simulink library "PCMULib"  (R2022b)
settings: Solver=ode45  StartTime=0.0  StopTime=10.0  RelTol=1e-3  EnableMultiTasking=on
undefined symbols (not defined in the file or in its folder): BreakpointData, BreakpointData1, BreakpointData2, BreakpointData_One_A, BreakpointData_Two_A, caaaa_dbi, caaaa_swi, cTmComprCtrl_n_i16SM4CmpHeatKiMax, cTmComprCtrl_n_i16SM4CmpHeatKiMin, cTmComprCtrl_n_i16SM4CmpHeatKpMax, cTmComprCtrl_n_i16SM4CmpHeatKpMin, cTmComprCtrl_Te_s32ErrCmpPIContinueHeatH, cTmComprCtrl_Te_s32ErrCmpPIContinueHeatL, cTmIn_n_ElacCmprReq_db, cTmIn_n_ElacCmprReq_sw, db, dbi, E2E_P01DataIDMode, E2E_P01ReceiverStatusType, EnumClass, iBit, initalValue, No_Runnable_Period, ObB_EidBsgStDerat_C, p_OVERRIDE_MASTER_SWITCH, SlDemoSign, sw, swi, SwitchOff_P, SwitchOn_P, Table, TableData_M, VCCTi33, VSysD_FidVehDerat1_C
libraries: simulink x22, CCMLib x11, simulink_need_slupdate x9, UXFD_Lib x7, canmsglib x2, PTCC_Lib x1, hdlsllib x1
(part 1 of 7)
settings Model: Creator=yaqi.zheng  LastModifiedBy=blue.ge
settings SolverCC: AlgebraicLoopSolver=TrustRegion
settings DataIOCC: LimitDataPoints=on  ReturnWorkspaceOutputs=off
settings OptimizationCC: LifeSpan=inf
settings DebuggingCC: UnconnectedInputMsg=warning  UnconnectedOutputMsg=warning  UnconnectedLineMsg=warning  AllowSymbolicDim=off  SFUnexpectedBacktrackingDiag=warning  SFNoUnconditionalDefaultTransitionDiag=warning  SFMachineParentedDataDiag=warning  ArithmeticOperatorsInVariantConditions=warning
settings ModelReferenceCC: EnableRefExpFcnMdlSchedulingChecks=on
settings SFSimCC: SimUseLocalCustomCode=off  CustomCodeUndefinedFunction=UseInterfaceOnly
settings RTWCC: RTWUseLocalCustomCode=off
settings CodeAppCC: StateflowObjectComments=on
settings GRTTargetCC: TargetLangStandard=C89/C90 (ANSI)
settings ConfigComp: CovMetricSettings=dw  CovSaveCumulativeToWorkspaceVar=on  CovSaveSingleToWorkspaceVar=on  CovExternalEMLEnable=off

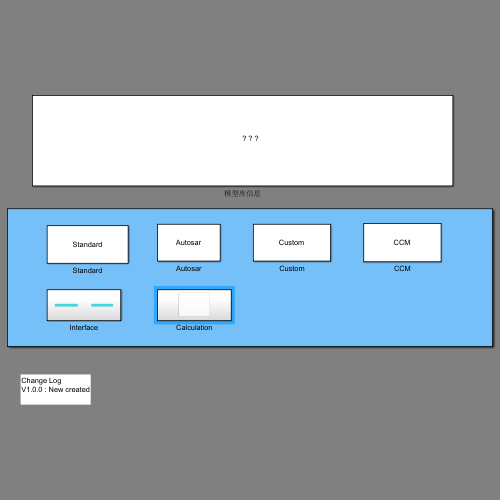
[thumbnail: Simulink's stored preview of the top-level diagram]
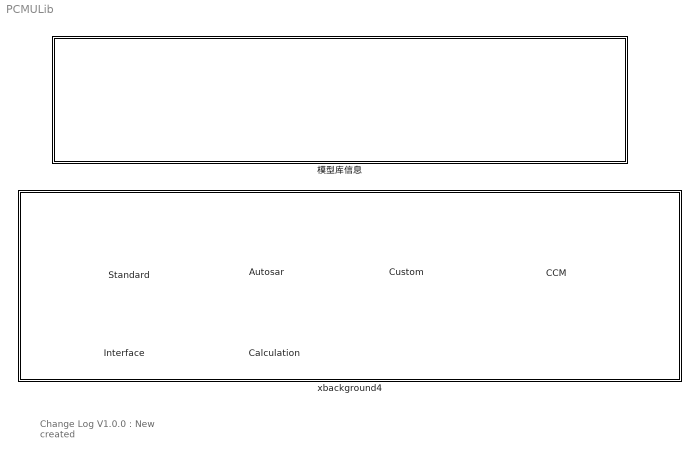
== system PCMULib ==
  note: Change Log
      | V1.0.0 : New created
  Autosar : Subsystem
      mask Display: disp('Autosar')
  CCM : Subsystem
      mask Display: disp('CCM')
  Calculation : Subsystem
  Custom : Subsystem
      mask Display: disp('Custom')
  Interface : Subsystem
  Standard : Subsystem
      mask Display: disp('Standard')
  xbackground4 : Subsystem
      mask Display: disp(' ')
  模型库信息 : Subsystem  mask(ModelHeader){prj=PCMU, desc=PCMU 模型库, ver=1.0.0, date=2023-10-11, rev=0, author=Blue, matlabver=MATLAB 2022b Version 9.13, simulinkver=MATLAB 2022b Version 10.6, stateflowver=MATLAB 2022b Version 10.7}
      mask prompts: prj "Project"; desc "Description"; ver "Version"; matlabver "MATLAB Ver"; simulinkver "Simulink Ver"; stateflowver "Stateflow Ver"
      mask init:
      | set_param(gcb, 'LinkStatus', 'none');
      mask Display:
      | plot([0 0 1 1 0],[0.03 1 1 0.03 0.03]) % 内层方框
      | plot([0.5 1],[0.85 0.85]) % 第一条横线
      | plot([0.5 1],[0.7 0.7]) % 第二条横线
      | plot([0.5 1],[0.55 0.55]) % 第三条线横线
      | plot([0.5 1],[0.4 0.4]) % 第四条线横线
      | plot([0 1],[0.25 0.25]) % 第五条横线
      | 
      | plot([0.5 0.5],[0.25 1]) % 第一条竖线
      | plot([0.60 0.60],[0.25 1])% 第二条竖线
      | plot([0.75 0.75],[0.25 1]) % 第三条竖线
      | plot([0.84 0.84],[0.25 1])% 第四条竖线
      | image(imread('geely.png','png'),[0.16 0.33 0.15 0.53]) % 图形位置
      | 
      | text(0.51,0.96,['\fontsize{8}\fontname{Times}\bfProject:'],'verticalAlignment','Top','horizontalAlignment','Left','texmode','on');
      | text(0.62,0.96,['\fontsize{8}\fontname{Times}\rm\fontsize{9}\fontsize{9}' prj],'verticalAlignment','Top','horizontalAlignment','Left','texmode','on');
      | 
      | text(0.51,0.81,['\fontsize{8}\fontname{Times}\bfVersion:' ],'verticalAlignment','Top','horizontalAlignment','Left','texmode','on');
      | text(0.62,0.81,['\fontsize{8}\fontname{Times}' ver],'verticalAlignment','Top','horizontalAlignment','Left','texmode','on');
      | 
      | text(0.51,0.67,['\fontsize{8}\fontname{Times}\bfDate:' ],'verticalAlignment','Top','horizontalAlignment','Left','texmode','on');
      | text(0.62,0.67,['\fontsize{8}\fontname{Times}\rm\fontsize{9}\fontsize{9}' date],'verticalAlignment','Top','horizontalAlignment','Left','texmode','on');
      | 
      | text(0.51,0.51,['\fontsize{8}\fontname{Times}\bfMATLAB Ver:' ],'verticalAlignment','Top','horizontalAlignment','Left','texmode','on');
      | text(0.62,0.51,['\fontsize{8}\fontname{Times}\rm\fontsize{9}\fontsize{9}' matlabver],'verticalAlignment','Top','horizontalAlignment','Left','texmode','on');
      | 
      | text(0.51,0.36,['\fontsize{8}\fontname{Times}\bfStateflow Ver:'],'verticalAlignment','Top','horizontalAlignment','Left','texmode','on');
      | text(0.62,0.36,['\fontsize{8}\fontname{Times}\rm\fontsize{9}\fontsize{9}' stateflowver],'verticalAlignment','Top','horizontalAlignment','Left','texmode','on');
      | %---------------------------------------------------------------------------------
      | text(0.76,0.96,['\fontsize{8}\fontname{Times}\bfAuthor:'],'verticalAlignment','Top','horizontalAlignment','Left','texmode','on');
      | text(0.86,0.96,['\fontsize{8}\fontname{Times}\rm\fontsize{9}\fontsize{9}' author],'verticalAlignment','Top','horizontalAlignment','Left','texmode','on');
      | 
      | text(0.76,0.81,['\fontsize{8}\fontname{Times}\bfRev:'],'verticalAlignment','Top','horizontalAlignment','Left','texmode','on');
      | text(0.86,0.81,['\fontsize{8}\fontname{Times}\rm\fontsize{9}\fontsize{9}' rev],'verticalAlignment','Top','horizontalAlignment','Left','texmode','on');
      | 
      | text(0.76,0.67,['\fontsize{8}\fontname{Times}\bfModel:'],'verticalAlignment','Top','horizontalAlignment','Left','texmode','on');
      | text(0.86,0.67,['\fontsize{8}\fontname{Times}\rm\fontsize{9}\fontsize{9}' desc],'verticalAlignment','Top','horizontalAlignment','Left','texmode','on');
      | 
      | text(0.76,0.51,['\fontsize{8}\fontname{Times}\bfSimulink Ver:'],'verticalAlignment','Top','horizontalAlignment','Left','texmode','on');
      | text(0.86,0.51,['\fontsize{8}\fontname{Times}\rm\fontsize{9}\fontsize{9}' simulinkver],'verticalAlignment','Top','horizontalAlignment','Left','texmode','on');
      | 
      | text(0.01,0.23,['\fontsize{8}\fontname{Times}\bfPROPRIETARY AND CONFIDENTIAL:\rm\fontsize{9}\newline\it\fontsize{10}\fontname{Arial}'                 'Geely Automobile Research Institute. All Right Reserved.'                 ],'verticalAlignment','Top','horizontalAlignment','Left','texmode','on');

== system PCMULib/Autosar ==
  note: Standard Core API AUTOSAR
  note: Advanced Core API AUTOSAR - use only if you know what you are doing
  note: E2E DEMO
  Constant6 : Constant  Value=72  OutDataTypeStr=Inherit: Inherit via back propagation
      settings: CopyFcn=set_param(gcbh,'ShowName','off');
  Constant7 : Constant  Value=220  OutDataTypeStr=Inherit: Inherit via back propagation
      settings: CopyFcn=set_param(gcbh,'ShowName','off');
  Dem_RepIUMPRDenLock : Subsystem  mask(Dem_RepIUMPRDenLock){}
      mask help: When enabled, this block will block the incrementation the denominator for Ratio Id Vc09XXXX.
      settings: AttributesFormatString=Dem_RepIUMPRDenLock
  Dem_RepIUMPRDenLock1 : PTCC_Lib/Autosar/Dem_RepIUMPRDenLock
      settings: AttributesFormatString=Dem_RepIUMPRDenLock
  Dem_RepIUMPRDenRelease : Subsystem  mask(Dem_RepIUMPRDenRelease){}
      mask help: When enabled, this block will release the incrementation the denominator for Ratio Id Vc09XXXX (i.e. if the conditions are fullfilled for incrementing the denominator for Ratio Id Vc09XXXX, it will be incremented).
      settings: AttributesFormatString=Dem_RepIUMPRDenRelease
  Dem_RepIUMPRFaultDetect : Subsystem  mask(Dem_RepIUMPRFaultDetect){}
      mask help: When enabled, report to the Core BSW, that Ratio Id Vc09XXXX has been able to detect a fault (increment Numerator for Ratio Id Vc09XXXX)
      settings: AttributesFormatString=Dem_RepIUMPRFaultDetect
  Dem_SetDTR : Subsystem  Description="API method to update mode $06 testdata.                                       Dem_SetDTR(UInt16 DTRId, sint32 TestVal, sint32 LowerLimit, sint32  UpperLimit, Ctrlval )"  mask(Vcc_SetDTR){lsb=1.0, offset=0}
      mask help:
      | Reports a DTR result with lower and upper limit.
      | The types of the TestValue and it limits should be Float32.
      | The test value and test limits are converted to Int32s using the
      | lsb and offset parameters in this block
      |
      | API is needed in OBD-relevant ECUs only
      settings: AttributesFormatString=Vcc_SetDTR
  Dem_SetEventStatusDepPF : Subsystem  TreatAsAtomicUnit=on  mask(Dem_SetEventStatusDepPre-Failed){}
      mask help:
      | Only to be used by dependability functions.
      | When enabled, events with status Pre-Failed is sent to the Diagnostic Core
      settings: AttributesFormatString=Dem_SetEventStatusDep\nPre-Failed
  Dem_SetEventStatusDepPP : Subsystem  TreatAsAtomicUnit=on  mask(Dem_SetEventStatusDepPre-Passed){}
      mask help:
      | Only to be used by dependability functions.
      | When enabled, events with status Pre-Passed is sent to the Diagnostic Core
      settings: AttributesFormatString=Dem_SetEventStatusDep\nPre-Passed
  Dem_SetEventStatusF : Subsystem  TreatAsAtomicUnit=on  mask(Dem_SetEventStatusFailed){}
      mask help: When enabled, events with status Failed is sent to the Diagnostic Core
      settings: AttributesFormatString=Dem_SetEventStatus\nFailed
  Dem_SetEventStatusP : Subsystem  mask(Dem_SetEventStatusPassed){}
      mask help: When enabled, events with status Passed is sent to the Diagnostic Core
      settings: AttributesFormatString=Dem_SetEventStatus\nPassed
  Dem_SetEventStatusPF : Subsystem  mask(Dem_SetEventStatusPre-Failed){}
      mask help: When enabled, events with status Pre-Failed is sent to the Diagnostic Core
      settings: AttributesFormatString=Dem_SetEventStatus\nPre-Failed
  Dem_SetEventStatusPP : Subsystem  mask(Dem_SetEventStatusPre-Passed){}
      mask help: When enabled, events with status Pre-Passed is sent to the Diagnostic Core
      settings: AttributesFormatString=Dem_SetEventStatus\nPre-Passed
  E2E_P01Protect : Subsystem
  E2E_P01_Check : Subsystem
  FiM_GetFunctionPermission : Subsystem  mask(FiM_GetFunctionPermission){}
      mask help:
      | When enabled, this block ask the core for permission to execute a monitor with the FID.
      | Note: If this is used for activating reconfigurations, Perm == 0 => Activate reconfiguration.
      settings: AttributesFormatString=FiM_GetFunctionPermission
  NamedConstant : Subsystem  mask(NamedConstant){const_name=VcEvName}
      mask prompts: const_name "Constant Name"
      mask help:
      | Enter a name for a preprocessor defined constant.
      | The following naming convention shall be used:
      | These prefixes shall be used for the following IDs (without underscores):
      | VcEv - Event IDs
      | VcFi - Function IDs (FiD)
      | VcRv - Ranking Value IDs
      | Vc06 - Mode $06 Test result IDs
      | Vc09 - IU(M)PR IDs (Mode $09)
      |
      | E.g.
      | VcEvBoostHigh - An event ID name for too high boost pressure
      | VcFiBoostPeak - A FiD for the Peak pressure boost monitor
      settings: AttributesFormatString=Named Constant
      mask Display: text(0.5, 0.5, get_param(gcb, 'const_name'), 'horizontalAlignment', 'center')
  Terminator7 : Terminator
  xbackground1 : UXFD_Lib/Autosar/xbackground4  SystemSampleTime=-1  VariantActivationTime=update diagram  Latency=0  AutoFrameSizeCalculation=off
  xbackground4 : Subsystem
      mask Display: disp(' ')
  xbackground5 : Subsystem
      mask Display: disp(' ')
  wires:
  E2E_P01Protect/1(E2E_P01Protect_ReturnType) -> Terminator7/1
  Constant6/1 -> E2E_P01Protect/1(DataLength)
  Constant7/1 -> E2E_P01Protect/2(DataID)

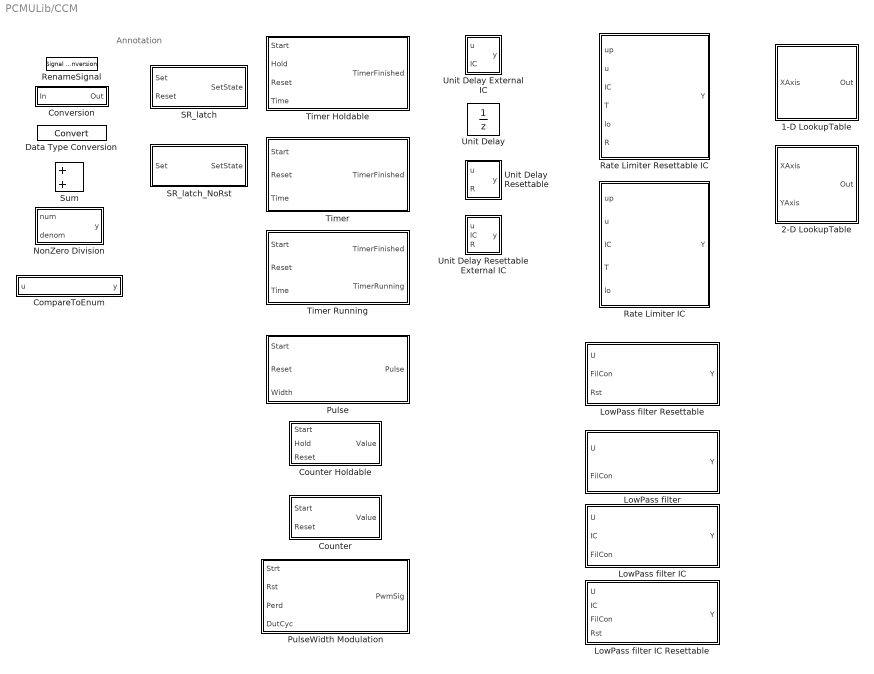
== system PCMULib/CCM ==
  note: Annotation
  1-D LookupTable : Subsystem  mask(1D Lookup table NGCC v1.1){TableData=[4 7 6], TableDataDataType=Inherit: auto, BreakpointsXAxis=[1:3], BreakpointsXAxisDataType=Inherit: auto}
      mask help:
      | NGCC version of the Simulink standard 2-D lookup table.
      | "X-axis" is used as notation instead of "breakpoints 1".
      | Deviation from standard 2-D lookup table default settings:
      | - Extrapolation method: Clip, use last table value for inputs at or above last breakpoint.
      | - Saturate on integer overflow.
      | - Integer rounding mode: Floor
      | - Does NOT require all inputs to have the same data type
      |
      | Mx-VDev tested: Yes
      mask init:
      | blkNameMask = gcb;
      | 
      | % Redraw block at resize
      | set_param(blkNameMask,'MaskRunInitForIconRedraw','on')
      mask Display:
      | pos = get_param(gcb, 'Position');
      | width = pos(3) - pos(1);
      | height = pos(4) - pos(2);
      | doPlot = true;
      | blockHandle = gcb;
      | try
      |     tableDialogText = get_param(blockHandle,'TableData');
      |     try
      |         table = evalin('base',tableDialogText);
      |         tableValue = table.Value;
      |     catch
      |         tableValue = recursiveMaskParameterSearch(blockHandle,tableDialogText);
      |     end
      |     breakpointsXAxisDialogText = get_param(blockHandle,'BreakpointsXAxis');
      |     try
      |         breakpointsXAxisHandle = evalin('base',breakpointsXAxisDialogText);
      |         bp1 = breakpointsXAxisHandle.Value;
      |     catch
      |         bp1 = recursiveMaskParameterSearch(blockHandle,breakpointsXAxisDialogText);
      |     end
      | catch
      |     tableValue = str2num(get_param(blockHandle,'TableData'));
      |     bp1 = str2num(get_param(blockHandle,'BreakpointsXAxis'));
      |     doPlot = true;
      |     if (isempty(tableValue) || isempty(bp1))
      |         doPlot = false;
      |     end
      | end
      | if doPlot
      |     % Scale table and breakpoint data to fit block icon size
      |     if min(tableValue(:)) == max(tableValue(:))
      |         tableScaleTemp2 = ones(size(tableValue))*10;
      |     else
      |         tableScaleTemp1 = tableValue-min(tableValue(:));
      |         tableScaleTemp2 = (tableScaleTemp1/(max(tableScaleTemp1(:))-min(tableScaleTemp1(:))))*((height-5)-10);
      |     end
      |     tableScaled = tableScaleTemp2 + 5;
      | 
      |     if min(bp1(:)) == max(bp1(:))
      |         bp1ScaleTemp2 = bp1;
      |     else
      |         bp1ScaleTemp1 = bp1-min(bp1(:));
      |         bp1ScaleTemp2 = (bp1ScaleTemp1/(max(bp1ScaleTemp1(:))-min(bp1ScaleTemp1(:))))*((width-5)-12);
      |     end
      |     bp1Scaled = bp1ScaleTemp2 + 12;
      | 
      |     % plot data
      |     for i=1:length(tableValue(:,1))
      |         try
      |             plot(bp1Scaled,tableScaled(i,:))
      |         catch
      |             disp(num2str(tableScaled(i,:)))
      |         end
      |     end
      | 
      | else
      |     disp('Input data\nError')
      | end
      | % plot axis
      | plot([12 12],[5 height-10])
      | plot([12 width-5],[5 5])
      | 
      | port_label('input',1,'X')
      | text(width/2-20,height-7,'1-D T(x)')
  2-D LookupTable : Subsystem  mask(2D Lookup table NGCC v1.1){TableData=[4 5 6;16 19 20;10 18 23], TableDataDataType=Inherit: auto, BreakpointsXAxis=[1:3], BreakpointsXAxisDataType=Inherit: auto, BreakpointsYAxis=[1:3], BreakpointsYAxisDataType=Inherit: auto}
      mask help:
      | NGCC version of the Simulink standard 2-D lookup table.
      | "X- and Y-axis" is used as notation instead of "breakpoints 1" and "breakpoints 2".
      | Deviation from standard 2-D lookup table default settings:
      | - Extrapolation method: Clip, use last table value for inputs at or above last breakpoint.
      | - Saturate on integer overflow.
      | - Integer rounding mode: Floor
      | - Does NOT require all inputs to have the same data type
      |
      | Mx-VDev tested: Yes
      mask init:
      | blkNameMask = gcb;
      | 
      | % Redraw block at resize
      | set_param(blkNameMask,'MaskRunInitForIconRedraw','on')
      mask Display:
      | pos = get_param(gcb, 'Position');
      | width = pos(3) - pos(1);
      | height = pos(4) - pos(2);
      | doPlot = true;
      | blockHandle = gcb;
      | try
      |     tableDialogText = get_param(blockHandle,'TableData');
      |     try
      |         table = evalin('base',tableDialogText);
      |         tableValue = table.Value;
      |     catch
      |         tableValue = recursiveMaskParameterSearch(blockHandle,tableDialogText);
      |     end
      |     breakpointsYAxisDialogText = get_param(blockHandle,'BreakpointsYAxis');
      |     try
      |         breakpointsYAxisHandle = evalin('base',breakpointsYAxisDialogText);
      |         bp2 = breakpointsYAxisHandle.Value;
      |     catch
      |         bp2 = recursiveMaskParameterSearch(blockHandle,breakpointsYAxisDialogText);
      |     end
      |     breakpointsXAxisDialogText = get_param(blockHandle,'BreakpointsXAxis');
      |     try
      |         breakpointsXAxisHandle = evalin('base',breakpointsXAxisDialogText);
      |         bp1 = breakpointsXAxisHandle.Value;
      |     catch
      |         bp1 = recursiveMaskParameterSearch(blockHandle,breakpointsXAxisDialogText);
      |     end
      | catch
      |     tableValue = str2num(get_param(blockHandle,'TableData'));
      |     bp2 = str2num(get_param(blockHandle,'BreakpointsYAxis'));
      |     bp1 = str2num(get_param(blockHandle,'BreakpointsXAxis'));
      |     doPlot = true;
      |     if (isempty(tableValue) || isempty(bp1) || isempty(bp2))
      |         doPlot = false;
      |     end
      | end
      | if doPlot
      |     % Scale table and breakpoint data to fit block icon size
      |     if min(tableValue(:)) == max(tableValue(:))
      |         tableScaleTemp2 = ones(size(tableValue))*10;
      |     else
      |         tableScaleTemp1 = tableValue-min(tableValue(:));
      |         tableScaleTemp2 = (tableScaleTemp1/(max(tableScaleTemp1(:))-min(tableScaleTemp1(:))))*((height-5)-10);
      |     end
      |     tableScaled = tableScaleTemp2 + 5;
      | 
      |     if min(bp1(:)) == max(bp1(:))
      |         bp1ScaleTemp2 = bp1;
      |     else
      |         bp1ScaleTemp1 = bp1-min(bp1(:));
      |         bp1ScaleTemp2 = (bp1ScaleTemp1/(max(bp1ScaleTemp1(:))-min(bp1ScaleTemp1(:))))*((width-5)-12);
      |     end
      |     bp1Scaled = bp1ScaleTemp2 + 12;
      | 
      |     % plot data
      |     for i=1:length(tableValue(:,1))
      |         try
      |             plot(bp1Scaled,tableScaled(i,:))
      |         catch
      |             disp(num2str(tableScaled(i,:)))
      |         end
      |     end
      | 
      | else
      |     disp('Input data\nError')
      | end
      | % plot axis
      | plot([12 12],[5 height-10])
      | plot([12 width-5],[5 5])
      | 
      | port_label('input',1,'X')
      | port_label('input',2,'Y')
      | text(width/2-20,height-7,'2-D T(x,y)')
  CompareToEnum : Subsystem  mask(Compare to Enum NGCC v1.0){relop===, const=EnumClass.Value, OutDataTypeStr=boolean, ZeroCross=on}
      mask prompts: relop "Simulink:masks:Operator_MP"; const "Simulink:masks:ConstantValue_MP"; OutDataTypeStr "Simulink:masks:OutputDataType_MP"; ZeroCross "Simulink:masks:EnableZerocrossingDetection_MP"
      mask help:
      | Compare to an Enum. Enum class is hidden from the mask i.e. displays only the value if the Enum is defined.
      |
      | Mx-VDev tested: Yes
      mask init:
      | blkName = gcb;
      | 
      | if strcmp(get_param(gcbh,'OutDataTypeStr'),'boolean')
      | 	setValue = 'boolean';
      | else
      | 	setValue = 'fixdt(0, 8)';
      | end
      | 
      | set_param([blkName,'/Compare'],'relop',relop, ...
      | 	'OutDataTypeStr', setValue, 'ZeroCross', ZeroCross);
      | 
      | str = [relop,' C']; %default
      | 
      | const_str = get_param(blkName, 'const');
      | 
      | if isempty(strfind(const_str, ' ')) && isempty(strfind(const_str, ','))
      |     % scalar or single expression
      |     if isempty(str2num(const_str))
      |         %expression
      |         str = [relop, ' ', const_str];
      |     elseif length(const) == 1
      |         if ismethod(const,'addClassNameToEnumNames') % Enum
      |             str = [relop,' ',char(const)];
      |         else
      |             str = [relop,' ',num2str(double(const))];
      |         end
      |     end
      | end
      mask TypeOptions relop: == | ~= | < | <= | >= | >
      mask TypeOptions OutDataTypeStr: uint8 | boolean
      mask Callback ZeroCross: sl('zeroCrossEnable', gcbh);
      mask Display: disp(str)
  Conversion : Subsystem  mask(Data Type Conversion NGCC v1.1){outputDataType=Inherit: Inherit via back propagation}
      mask prompts: outputDataType "Convert data type to:"
      mask help:
      | CCM version of the standard Simulink block.
      | This version displays the output data type name on the block icon, regardless of data type.
      |
      | Mx-VDev tested: Yes
      mask Display:
      | if strcmp(char(get_param(gcb,'MaskValues')),'Inherit: Inherit via back propagation')
      |     disp('Conversion')
      | else
      |     disp(char(get_param(gcb,'MaskValues')))
      | end
  Counter : Subsystem  mask(Counter NGCC v1.0){}
      mask help:
      | If Start (1) is true, the counter is started.
      | Counter will be reset to 0 and stopped if Reset (2) is true.
      | This block is reset dominant.
      | Value (output) specifies the counter value, data type VCCUInt32.
      |
      | Mx-VDev tested: Yes
      mask Display:
      | try
      |     image(imread([CCMConfig.GetRootDir '\Shared\SimulinkLibrary\Images\counter.bmp']))
      | catch
      |     fprintf('Counter\nHoldable')
      | end
      | port_label('output',1,'Value')
      | port_label('input',1,'Start')
      | port_label('input',2,'Reset')
  Counter Holdable : Subsystem  mask(Counter Holdable NGCC v1.0){}
      mask help:
      | If Start (1) is true, the counter is started.
      | Counter will continue counting until Hold (2) is true, then the counter value will be held.
      | Counter will be reset to 0 if Reset (3) is true.
      | Value (output) specifies the counter value, data type VCCUInt32.
      |
      | Mx-VDev tested: Yes
      mask Display:
      | try
      |     image(imread([CCMConfig.GetRootDir '\Shared\SimulinkLibrary\Images\counter.bmp']))
      | catch
      |     fprintf('Counter\nHoldable')
      | end
      | port_label('output',1,'Value')
      | port_label('input',1,'Start')
      | port_label('input',2,'Hold')
      | port_label('input',3,'Reset')
  Data Type Conversion : DataTypeConversion  RndMeth=Floor
      settings: AttributesFormatString=%<OutDataTypeStr>
  LowPass filter : Subsystem  mask(Low-pass filter NGCC v1.0){InputOutputDataType=single, FilterConstantDataType=VCCTi33, RunnablePeriod=No_Runnable_Period}
      mask prompts: InputOutputDataType "Input/Output Data Type"; FilterConstantDataType "Filter Time Constant Data Type:"; RunnablePeriod "SWC Sampling Time Parameter:"
      mask help:
      | Typical NGCC low-pass filter with filter length 1.
      | U is the input signal that is to be filtered.
      | FilCon is the filter time constant.
      | Y is the filtered output.
      |
      | Mx-VDev tested: Yes
      mask init:
      | blkNameMask = gcb;
      | IODataType = get_param(blkNameMask,'InputOutputDataType');
      | if strcmp(IODataType,'single')
      |     dataTypeSlope = 2^(-12);
      | else
      |     try
      |     dataTypeSlope = evalin('base',[IODataType '.Slope']); %Fixed point
      |     catch
      |         dataTypeSlope = 1; %Integer
      |     end
      | end
      | %Set sampletime
      | blkName = gcb;
      | modelName = char(regexp(blkName,'(\w*)_(?:Runnable|lib)','tokens','once'));
      | if isempty(modelName)
      |     modelName = 'No';
      | end
      | timeParameter = [modelName '_Runnable_Period'];
      | set_param(blkName, 'RunnablePeriod',timeParameter);
      mask Display: disp(['Y = U[n]*k + Y[n-1]*(1-k)' char(uint16(10)) 'n: sample' char(uint16(10)) 'k: filter constant' char(uint16(10)) 'Init value = U[0]']);
  LowPass filter Resettable : Subsystem  mask(Low-pass filter Resettable NGCC v1.0){InputOutputDataType=single, FilterConstantDataType=VCCTi33, RunnablePeriod=No_Runnable_Period}
      mask prompts: InputOutputDataType "Input/Output Data Type"; FilterConstantDataType "Filter Time Constant Data Type:"; RunnablePeriod "SWC Sampling Time Parameter:"
      mask help:
      | Typical NGCC low-pass filter with filter length 1.
      | U is the input signal that is to be filtered.
      | FilCon is the filter time constant.
      | Rst is the filter reset condition (boolean).
      | Y is the filtered output.
      |
      | Mx-VDev tested: Yes
      mask init:
      | %Set sample time
      | blkName = gcb;
      | modelName = char(regexp(blkName,'(\w*)_(?:Runnable|lib)','tokens','once'));
      | if isempty(modelName)
      |     modelName = 'No';
      | end
      | timeParameter = [modelName '_Runnable_Period'];
      | set_param(blkName, 'RunnablePeriod',timeParameter);
      mask Display: disp(['Y = U[n]*k + Y[n-1]*(1-k)' char(uint16(10)) 'n: sample' char(uint16(10)) 'k: filter constant' char(uint16(10)) 'Init value = U[0]']);
  LowPass filter IC : Subsystem  mask(Low-pass filter IC NGCC v1.0){InputOutputDataType=single, FilterConstantDataType=VCCTi33, RunnablePeriod=No_Runnable_Period}
      mask prompts: InputOutputDataType "Input/Output Data Type"; FilterConstantDataType "Filter Time Constant Data Type:"; RunnablePeriod "SWC Sampling Time Parameter:"
      mask help:
      | Typical NGCC low-pass filter with filter length 1.
      | U is the input signal that is to be filtered.
      | IC is the initial condition value.
      | FilCon is the filter time constant.
      | Y is the filtered output.
      |
      | Mx-VDev tested: No
      mask init:
      | blkNameMask = gcb;
      | IODataType = get_param(blkNameMask,'InputOutputDataType');
      | if strcmp(IODataType,'single')
      |     dataTypeSlope = 2^(-12);
      | else
      |     try
      |     dataTypeSlope = evalin('base',[IODataType '.Slope']); %Fixed point
      |     catch
      |         dataTypeSlope = 1; %Integer
      |     end
      | end
      | 
      | %Set sample time
      | blkName = gcb;
      | modelName = char(regexp(blkName,'(\w*)_(?:Runnable|lib)','tokens','once'));
      | if isempty(modelName)
      |     modelName = 'No';
      | end
      | timeParameter = [modelName '_Runnable_Period'];
      | set_param(blkName, 'RunnablePeriod',timeParameter);
      mask Display: disp(['Y = U[n]*k + Y[n-1]*(1-k)' char(uint16(10)) 'n: sample' char(uint16(10)) 'k: filter constant' char(uint16(10)) 'Init value = IC']);
  LowPass filter IC Resettable : Subsystem  mask(Low-pass filter IC Resettable NGCC v1.0){InputOutputDataType=single, FilterConstantDataType=VCCTi33, RunnablePeriod=No_Runnable_Period}
      mask prompts: InputOutputDataType "Input/Output Data Type"; FilterConstantDataType "Filter Time Constant Data Type:"; RunnablePeriod "SWC Sampling Time Parameter:"
      mask help:
      | Typical NGCC low-pass filter with filter length 1.
      | IC is the initial condition (value).
      | U is the input signal that is to be filtered.
      | FilCon is the filter time constant.
      | Rst is the filter reset condition (boolean).
      | Y is the filtered output.
      |
      | Mx-VDev tested: No
      mask init: same as PCMULib/CCM/LowPass filter Resettable
      mask Display: disp(['Y = U[n]*k + Y[n-1]*(1-k)' char(uint16(10)) 'n: sample' char(uint16(10)) 'k: filter constant' char(uint16(10)) 'Init value = IC']);
  NonZero Division : Subsystem  mask(Non Zero Division NGCC v1.3){dataTypeNum=single, dataTypeDen=single, dataTypeOut=single}
      mask prompts: dataTypeNum "Data type of numerator"; dataTypeDen "Data type of denominator"; dataTypeOut "Data type of output"
      mask help:
      | Performs a division that is protected against division by zero.
      | First input is numerator, second input is denominator.
      | User must enter the data types of the two input signals as well as the output signal.
      |
      | Mx-VDev tested: Yes
      mask init:
      | blkNameMask = gcb;
      | DenominatorDataType = get_param(blkNameMask,'dataTypeDen');
      | if strcmp(DenominatorDataType,'single')
      |     dataTypeSlope = 2^(-100);
      | else
      |     try
      |         dataTypeSlope = evalin('base',[DenominatorDataType '.Slope']); %Fixed point
      |     catch
      |         dataTypeSlope = 1; %Integer
      |     end
      | end
      mask Display:
      | port_label('output',1,'y')
      | port_label('input',1,'x')
      | port_label('input',2,'÷')
      | fprintf('Non-Zero\nDivision')
  Pulse : Subsystem  mask(Pulse NGCC v1.0){timeDataType=VCCTi33, RunnablePeriod=No_Runnable_Period}
      mask prompts: timeDataType "Pulse width data type (s):"; RunnablePeriod "SWC Sampling Time Parameter:"
      mask help:
      | If Start (1) is true, the Pulse (output) is started.
      | If Start is set during [Pulse == true], the timer is reset and the Pulse is kept true.
      | Pulse will be reset to 0 if Reset (2) is true.
      | Width (3) defines the pulse width in seconds.
      | If Width is set to zero, Pulse will be set to false.
      | Reset is always master over Start.
      |
      | Mx-VDev tested: Yes
      mask init: same as PCMULib/CCM/LowPass filter Resettable
      mask Display:
      | x=[0.2 0.35 0.35 0.65 0.65 0.8];
      | y=[0.2 0.2 0.7 0.7 0.2 0.2];
      | plot(x,y)
  PulseWidth Modulation : Subsystem  mask(PulseWidth Modulation NGCC v1.0){timeDataType=VCCTi33, RunnablePeriod=No_Runnable_Period}
      mask prompts: timeDataType "Period time input data type:"; RunnablePeriod "SWC Sampling Time Parameter:"
      mask help:
      | If Start(1) is true the pulse generator is started.
      | It will continue to run until Reset(2) is true. It will start again when Reset is set to false.
      | Data type of Period time(3) and the SWC Sampling Time has to be specified in the mask.
      | Data type of Duty Cycle(4) is VCCPerc30 and determines the ratio of the period time when the signal is true.
      | The period starts with the duty cycle, i.e. the signal is first true after reset or start.
      | Default value, when pulse generator is not started or when it is held with the reset function, is true.
      |
      | Mx-VDev tested: Yes
      mask init: same as PCMULib/CCM/LowPass filter Resettable
      mask Display:
      | x=[0.1 1 1 2.1 2.1 3 3 4.1 4.1 5 5 6.1 6.1 7 7 8.1] * 10 + 30;
      | y=[1 1 0 0 1 1 0 0 1 1 0 0 1 1 0 0] * 15 + 30;
      | plot(x,y)
  Rate Limiter IC : Subsystem  mask(Rate Limiter Dynamic IC NGCC v1.0){InputOutputDataType=single}
      mask prompts: InputOutputDataType "Data type inputs/output:"
      mask help:
      | Limit rising and falling rates of the input signal.
      | up: upper rate limit
      | u: input signal to be rate limited
      | IC: initial condition
      | T: SWC runnable period
      | lo: lower rate limit (input should be negative)
      |
      | The rates 'up' and 'lo' should be per second (*/s), since the block converts seconds to sample before calculations.
      |
      | Mx-VDev tested: Yes
      mask Display: plot([0.15 0.95],[.5 .5],[.5 .5],[0.05 0.95],0.05+0.9*[.2 .8],0.05+0.9*[0 1]);
  Rate Limiter Resettable IC : Subsystem  mask(Rate Limiter Dynamic Resettable IC NGCC v1.0){InputOutputDataType=single}
      mask prompts: InputOutputDataType "Data type inputs/output:"
      mask help:
      | Limit rising and falling rates of the input signal.
      | up: upper rate limit
      | u: input signal to be rate limited
      | IC: initial condition
      | T: SWC runnable period
      | lo: lower rate limit
      | R: reset flag, resets to the initial condition
      |
      | The rates 'up' and 'lo' should be per second (*/s), since the block converts seconds to sample before calculations.
      |
      | Mx-VDev tested: Yes
      mask Display: plot([0.15 0.95],[.5 .5],[.5 .5],[0.05 0.95],0.05+0.9*[.2 .8],0.05+0.9*[0 1]);
  RenameSignal : SignalConversion  OverrideOpt=on  mask(Rename signal NGCC v1.1){}
      mask help:
      | Typically used when bus signals are relayed.
      |
      | Mx-VDev tested: Yes
      mask Display: fprintf('Rename')
  SR_latch : Subsystem  mask(SR-latch NGCC v1.0){}
      mask help:
      | Set/reset-latch with default value 0 (false).
      | S   R   Q
      | ----------
      | 0   0   Q[n-1]
      | 0   1   0
      | 1   0   1
      | 1   1   0
      |
      | where Q[n-1] is the previous output value.
      |
      | Mx-VDev tested: Yes
  SR_latch_NoRst : Subsystem  mask(SR-latch-no-reset NGCC v1.0){}
      mask help:
      | Set-latch with default value 0 (false).
      | S   Q
      | ----------
      | 0   Q[n-1]
      | 1   1
      |
      | where Q[n-1] is the previous output value.
      |
      | Mx-VDev tested: Yes
  Sum : Sum  InputSameDT=on  SaturateOnIntegerOverflow=on
  Timer : Subsystem  mask(Timer NGCC v1.0){timeDataType=VCCTi33, RunnablePeriod=No_Runnable_Period}
      mask prompts: timeDataType "Time data type:"; RunnablePeriod "SWC Sampling Time Parameter:"
      mask help:
      | If Start (1) is true, the timer is started.
      | The timer works as a "set/reset"-functionality, i.e. start does not have to be "true" continuously to keep the timer running.
      | Timer will be reset to 0 if Reset (2) is true.
      | TimerFinished (output) specifies if the timer is finished (boolean).
      | If Time (3) is set to zero, this block will function as a set-reset latch.
      | Reset is always master over Start.
      |
      | Mx-VDev tested: Yes
      mask init: same as PCMULib/CCM/LowPass filter Resettable
      mask Display:
      | try
      |     image(imread([CCMConfig.GetRootDir '\Shared\SimulinkLibrary\Images\timer.bmp']))
      | catch
      |     fprintf('Timer\nHoldable')
      | end
      | port_label('output',1,'TmrFinshd')
      | port_label('input',1,'Start')
      | port_label('input',2,'Reset')
      | port_label('input',3,'Time')
  Timer Holdable : Subsystem  mask(Timer Holdable NGCC v1.1){timeDataType=VCCTi33, RunnablePeriod=No_Runnable_Period}
      mask prompts: timeDataType "Time data type:"; RunnablePeriod "SWC Sampling Time Parameter:"
      mask help:
      | If Start (1) is true, the timer is started.
      | Timer will continue running until Hold (2) is true, then the timer value will be held.
      | If Hold becomes false, the timer will continue when conditions to start is fulfilled.
      | The Start and Hold serve as a "set/reset"-functionality, i.e. start does not have to be "true" continuously to keep the timer running.
      | Timer will be reset to 0 if Reset (3) is true.
      | TimerFinished (output) specifies if the timer is finished (boolean).
      | If Time is set to zero, this block will function as a set-reset latch.
      | Hold and Reset are always master over Start.
      |
      | Mx-VDev tested: Yes
      mask init: same as PCMULib/CCM/LowPass filter Resettable
      mask Display:
      | try
      |     image(imread([CCMConfig.GetRootDir '\Shared\SimulinkLibrary\Images\timer.bmp']))
      | catch
      |     fprintf('Timer\nHoldable')
      | end
      | port_label('output',1,'TmrFinshd')
      | port_label('input',1,'Start')
      | port_label('input',2,'Hold')
      | port_label('input',3,'Reset')
      | port_label('input',4,'Time')
  Timer Running : Subsystem  mask(Timer Running NGCC v1.0){timeDataType=VCCTi33, RunnablePeriod=No_Runnable_Period}
      mask prompts: timeDataType "Time data type:"; RunnablePeriod "SWC Sampling Time Parameter:"
      mask help:
      | If Start (1) is true, the timer is started.
      | The timer works as a "set/reset"-functionality, i.e. start does not have to be "true" continuously to keep the timer running.
      | Timer will be reset to 0 if Reset (2) is true.
      | TimerFinished (output) specifies if the timer is finished (boolean).
      | If Time (3) is set to zero, this block will function as a set-reset latch.
      | Reset is always master over Start.
      |
      | TmrRunng (output 2) will be set when timer is activated.
      |
      | Mx-VDev tested: Yes
      mask init: same as PCMULib/CCM/LowPass filter Resettable
      mask Display:
      | try
      |     image(imread([CCMConfig.GetRootDir '\Shared\SimulinkLibrary\Images\timer.bmp']))
      | catch
      |     fprintf('Timer\nHoldable')
      | end
      | port_label('output',1,'TmrFinshd')
      | port_label('output',2,'TmrRunng')
      | port_label('input',1,'Start')
      | port_label('input',2,'Reset')
      | port_label('input',3,'Time')
  Unit Delay : UnitDelay  InitialCondition=initalValue  SampleTime=-1  HasFrameUpgradeWarning=on
      settings: AttributesFormatString=X0=%<X0>
  Unit Delay External IC : Subsystem  mask(Unit Delay External Initial Condition NGCC v1.0){dataType=single}
      mask prompts: dataType "Data type:"
      mask help:
      | NGCC version of the Simulink built-in block with data type control and boolean datatype usage for internal switch condition.
      | -----------------------------------------------------
      | Normally, the output is the signal u delayed by one sample period.
      | The initial condition is given by the signal IC.
      |
      | Mx-VDev tested: Yes
      mask Display: dpoly(1,[1 0],'z')
  Unit Delay Resettable : Subsystem  mask(Unit Delay Resettable NGCC v1.0){initialCondition=0, dataType=single}
      mask prompts: initialCondition "Initial condition:"; dataType "Data type:"
      mask help:
      | NGCC version of the Simulink built-in block with data type control and boolean datatype usage for internal switch condition.
      | -----------------------------------------------------
      | Normally, the output is the signal u delayed by one sample period.
      | When the reset signal R is true, the state and the output are always set equal to the initial condition parameter.  This reset action is vectorized and supports scalar expansion.
      |
      | Mx-VDev tested: Yes
      settings: AttributesFormatString=X0=%<initialCondition>
      mask Display: dpoly(1,[1 0],'z')
  Unit Delay Resettable External IC : Subsystem  mask(Unit Delay Resettable External Initial Condition NGCC v1.0){dataType=single}
      mask prompts: dataType "Data type:"
      mask help:
      | NGCC version of the Simulink built-in block with data type control and boolean datatype usage for internal switch condition.
      | -----------------------------------------------------
      | Normally, the output is the signal u delayed by one sample period.
      | When the reset signal R is true, the state and the output are always set equal to the initial condition signal IC.  This reset action is vectorized and supports scalar expansion.
      |
      | Mx-VDev tested: Yes
      mask Display: dpoly(1,[1 0],'z')

== system PCMULib/Calculation ==
  PI : Subsystem
  interpolation : Subsystem

== system PCMULib/Custom ==
  CAN : Subsystem
      mask Display: disp('CAN')
  Diagnose : Subsystem
      mask Display: disp('Diagnose')
  PIN : Subsystem
      mask Display: disp('PIN')
  xbackground4 : UXFD_Lib/xbackground4  SystemSampleTime=-1  VariantActivationTime=update diagram  Latency=0  AutoFrameSizeCalculation=off

== system PCMULib/Interface ==
  Indebug : Subsystem  mask(Signal_In){SWI=swi, DBI=dbi}
      mask prompts: SWI "Debug_SWI:"; DBI "Debug_DBI:"
      mask help: Interface block to debug input signal.
      mask TypeOptions SWI: SWI/Value
      mask TypeOptions DBI: Debug_In/DBI/Value
      mask Display:
      | Name2 ='Nan';
      | finish = 0;
      | for i = 1:5
      |     if i == 1
      |         PortConn = get(gcbh,'PortConnectivity');
      |     else
      |         PortConn = get(Handle,'PortConnectivity');
      |     end
      |     DstBlk = PortConn(length(PortConn)).DstBlock;
      | 
      |     j=length(DstBlk);
      |     if j == 0
      |         break;
      |     else
      |         for k = 1:j
      |             if isequal(get(DstBlk(k),'BlockType'),'Outport')
      |                 Name2 = get(DstBlk(k),'Name');
      |                 finish = 1;
      |                 break;
      |             elseif isequal(get(DstBlk(k),'BlockType'),'SubSystem')
      |                 Handle = DstBlk(k);
      |                 break;
      |             end
      |         end
      |     end
      |     if finish ==1
      |         break;
      |     end
      | end
      | 
      | if isequal(Name2,'Nan')
      |     set(gcbh,'SWI','swi');
      |     set(gcbh,'DBI','dbi');
      | else
      |     set(gcbh,'SWI',['c' Name2(2:end) '_swi']);
      |     set(gcbh,'DBI',['c' Name2(2:end) '_dbi']);
      | end
      | 
      | text(0.55,0.86,sprintf('%s', Name2),...
      |     'horizontalAlignment','center',...
      |     'verticalAlignment', 'top');
  IndebugRvs : Subsystem  mask(Signal_In){SWI=caaaa_swi, DBI=caaaa_dbi}
      mask prompts: SWI "Debug_SWI:"; DBI "Debug_DBI:"
      mask help: Interface block to debug input signal.
      mask TypeOptions SWI: SWI/Value
      mask TypeOptions DBI: Debug_In/DBI/Value
      mask Display:
      | Name2 ='Nan';
      | finish = 0;
      | for i = 1:5
      |     if i == 1
      |         PortConn = get(gcbh,'PortConnectivity');
      |     else
      |         PortConn = get(Handle,'PortConnectivity');
      |     end
      |     SrcBlk = PortConn(1).SrcBlock;
      | 
      |     j=length(SrcBlk);
      |     if j == 0
      |         break;
      |     else
      |         for k = 1:j
      |             if isequal(get(SrcBlk(k),'BlockType'),'Inport')
      |                 Name2 = get(SrcBlk(k),'Name');
      |                 finish = 1;
      |                 break;
      |             elseif isequal(get(SrcBlk(k),'BlockType'),'SubSystem')
      |                 Handle = SrcBlk(k);
      |                 break;
      |             end
      |         end
      |     end
      |     if finish ==1
      |         break;
      |     end
      | end
      | 
      | if isequal(Name2,'Nan')
      |     set(gcbh,'SWI','swi');
      |     set(gcbh,'DBI','dbi');
      | else
      |     set(gcbh,'SWI',['c' Name2(2:end) '_swi']);
      |     set(gcbh,'DBI',['c' Name2(2:end) '_dbi']);
      | end
      | 
      | text(0.55,0.86,sprintf('%s', Name2),...
      |     'horizontalAlignment','center',...
      |     'verticalAlignment', 'top');
  Outdebug : Subsystem  mask(Signal_In){SWI=cTmIn_n_ElacCmprReq_sw, DBI=cTmIn_n_ElacCmprReq_db}
      mask prompts: SWI "Debug_SWI:"; DBI "Debug_DBI:"
      mask help: Interface block to debug input signal.
      mask TypeOptions SWI: SWI/Value
      mask TypeOptions DBI: Debug_In/DBI/Value
      mask Display:
      | Name2 ='Nan';
      | finish = 0;
      | for i = 1:5
      |     if i == 1
      |         PortConn = get(gcbh,'PortConnectivity');
      |     else
      |         PortConn = get(Handle,'PortConnectivity');
      |     end
      |     SrcBlk = PortConn.SrcBlock;
      | 
      |     j=length(SrcBlk);
      |     if j == 0
      |         break;
      |     else
      |         for k = 1:j
      |             if isequal(get(SrcBlk(k),'BlockType'),'Inport')
      |                 Name2 = get(SrcBlk(k),'Name');
      |                 finish = 1;
      |                 break;
      |             elseif isequal(get(SrcBlk(k),'BlockType'),'SubSystem')
      |                 Handle = SrcBlk(k);
      |                 break;
      |             end
      |         end
      |     end
      |     if finish ==1
      |         break;
      |     end
      | end
      | 
      | if isequal(Name2,'Nan')
      |     set(gcbh,'SWI','sw');
      |     set(gcbh,'DBI','db');
      | else
      |     set(gcbh,'SWI',['c' Name2(2:end) '_sw']);
      |     set(gcbh,'DBI',['c' Name2(2:end) '_db']);
      | end
      | 
      | text(0.55,0.86,sprintf('%s', Name2),...
      |     'horizontalAlignment','center',...
      |     'verticalAlignment', 'top');
      | port_label('input',1,'TmOut');
  OutdebugRvs : Subsystem  mask(Signal_In){SWI=sw, DBI=db}
      mask prompts: SWI "Debug_SWI:"; DBI "Debug_DBI:"
      mask help: Interface block to debug input signal.
      mask TypeOptions SWI: SWI/Value
      mask TypeOptions DBI: Debug_In/DBI/Value
      mask Display:
      | Name2 ='Nan';
      | finish = 0;
      | for i = 1:5
      |     if i == 1
      |         PortConn = get(gcbh,'PortConnectivity');
      |     else
      |         PortConn = get(Handle,'PortConnectivity');
      |     end
      |     DstBlk = PortConn(2).DstBlock;
      | 
      |     j=length(DstBlk);
      |     if j == 0
      |         break;
      |     else
      |         for k = 1:j
      |             if isequal(get(DstBlk(k),'BlockType'),'Outport')
      |                 Name2 = get(DstBlk(k),'Name');
      |                 finish = 1;
      |                 break;
      |             elseif isequal(get(DstBlk(k),'BlockType'),'SubSystem')
      |                 Handle = DstBlk(k);
      |                 break;
      |             end
      |         end
      |     end
      |     if finish ==1
      |         break;
      |     end
      | end
      | 
      | if isequal(Name2,'Nan')
      |     set(gcbh,'SWI','sw');
      |     set(gcbh,'DBI','db');
      | else
      |     set(gcbh,'SWI',['c' Name2(2:end) '_sw']);
      |     set(gcbh,'DBI',['c' Name2(2:end) '_db']);
      | end
      | 
      | text(0.55,0.86,sprintf('%s', Name2),...
      |     'horizontalAlignment','center',...
      |     'verticalAlignment', 'top');
      | port_label('input',1,'TmOut');

== system PCMULib/Standard ==
  Bit Operation : Subsystem
      settings: CopyFcn=set_param(gcbh,'ShowName','off');
      mask Display: disp('Bit Operation')
  Calibration : Subsystem
      settings: CopyFcn=set_param(gcbh,'ShowName','off');
      mask Display: disp('Calibration')
  Discrete dynamics : Subsystem
      settings: CopyFcn=set_param(gcbh,'ShowName','off');
      mask Display: disp('Discrete dynamics')
  Math : Subsystem
      mask Display: disp('Math')
  Relation&Logic : Subsystem
      mask Display: disp('Relation & Logic')
  Signals and systems : Subsystem
      mask Display: disp('Signals and systems')
  xbackground4 : UXFD_Lib/xbackground4  SystemSampleTime=-1  VariantActivationTime=update diagram  Latency=0  AutoFrameSizeCalculation=off

== system PCMULib/xbackground4 ==

== system PCMULib/模型库信息 ==

== system PCMULib/Autosar/Dem_RepIUMPRDenLock ==
  Vc09 : Inport
  EntryCond : EnablePort
  Dem_RepIUMPRDenLock : S-Function  FunctionName=Dem_RepIUMPRDenLock_flp  Parameters=dt  SFunctionDeploymentMode=off  EnableBusSupport=off  mask(TL_CustomCode){data={'#state',0,'#param',0,'#work',0,'codefile','Dem_RepIUMPRDenLock.c','prodcode',0,'logdata',{'plotchannels',[]},'output',{'name','$S_ok','varname','ok','type','Bool'},'input',{'name','$S_RatioId','varname','RatioId','type','UInt16'},'date',735300.29244876152}, dt=-1}
      mask help:
      | TargetLink Custom Code block:
      | Allows to insert custom code into a TargetLink application.
      settings: AttributesFormatString=Dem_RepIUMPRDenLock  DeleteFcn=if exist('delete_tlblock','file')==2,delete_tlblock(gcbh);end  NameChangeFcn=if exist('rename_tlblock','file')==2,rename_tlblock(gcbh);end  OpenFcn=if exist('tl_open_blockdlg','file')==2,tl_open_blockdlg(gcbh);else,open_system(gcbh,'mask');end
      mask Help: eval(['tl_online_help(''Topic'',''',get_param(gcbh,'MaskType'),''')'])
      mask Display:
      | plot([-0.05, 1.05, NaN, -0.05, 1.05],[.01, .01, NaN, .99, .99])
      | ; disp('Dem_RepIUMPRDenLock.c');port_label('input',1,'RatioId');port_label('output',1,'ok');
  Terminator3 : Terminator
  wires:
  Vc09/1 -> Dem_RepIUMPRDenLock/1
  Dem_RepIUMPRDenLock/1 -> Terminator3/1

== system PCMULib/Autosar/Dem_RepIUMPRDenRelease ==
  Vc09 : Inport
  EntryCond : EnablePort
  Dem_RepIUMPRDenRelease : S-Function  FunctionName=Dem_RepIUMPRDenRelease_flp  Parameters=dt  SFunctionDeploymentMode=off  EnableBusSupport=off  mask(TL_CustomCode){data={'#state',0,'#param',0,'#work',0,'codefile','Dem_RepIUMPRDenRelease.c','prodcode',0,'logdata',{'plotchannels',[]},'output',{'name','$S_ok','varname','ok','type','Bool'},'input',{'name','$S_RatioId','varname','RatioId','type','UInt16'},'date',735300.29243282403}, dt=-1}
      mask help:
      | TargetLink Custom Code block:
      | Allows to insert custom code into a TargetLink application.
      settings: AttributesFormatString=Dem_RepIUMPRDenRelease  DeleteFcn=if exist('delete_tlblock','file')==2,delete_tlblock(gcbh);end  NameChangeFcn=if exist('rename_tlblock','file')==2,rename_tlblock(gcbh);end  OpenFcn=if exist('tl_open_blockdlg','file')==2,tl_open_blockdlg(gcbh);else,open_system(gcbh,'mask');end
      mask Help: eval(['tl_online_help(''Topic'',''',get_param(gcbh,'MaskType'),''')'])
      mask Display:
      | plot([-0.05, 1.05, NaN, -0.05, 1.05],[.01, .01, NaN, .99, .99])
      | ; disp('Dem_RepIUMPRDenRelease.c');port_label('input',1,'RatioId');port_label('output',1,'ok');
  Terminator3 : Terminator
  wires:
  Dem_RepIUMPRDenRelease/1 -> Terminator3/1
  Vc09/1 -> Dem_RepIUMPRDenRelease/1

== system PCMULib/Autosar/Dem_RepIUMPRFaultDetect ==
  Vc09 : Inport
  EntryCond : EnablePort
  Dem_RepIUMPRFaultDetect : S-Function  FunctionName=Dem_RepIUMPRFaultDetect_flp  Parameters=dt  SFunctionDeploymentMode=off  EnableBusSupport=off  mask(TL_CustomCode){data={'#state',0,'#param',0,'#work',0,'codefile','Dem_RepIUMPRFaultDetect.c','prodcode',0,'logdata',{'plotchannels',[]},'output',{'name','$S_ok','varname','ok','type','Bool'},'input',{'name','$S_RatioId','varname','RatioId','type','UInt16'},'date',735300.29241528932}, dt=-1}
      mask help:
      | TargetLink Custom Code block:
      | Allows to insert custom code into a TargetLink application.
      settings: AttributesFormatString=Dem_RepIUMPRFaultDetect  DeleteFcn=if exist('delete_tlblock','file')==2,delete_tlblock(gcbh);end  NameChangeFcn=if exist('rename_tlblock','file')==2,rename_tlblock(gcbh);end  OpenFcn=if exist('tl_open_blockdlg','file')==2,tl_open_blockdlg(gcbh);else,open_system(gcbh,'mask');end
      mask Help: eval(['tl_online_help(''Topic'',''',get_param(gcbh,'MaskType'),''')'])
      mask Display:
      | plot([-0.05, 1.05, NaN, -0.05, 1.05],[.01, .01, NaN, .99, .99])
      | ; disp('Dem_RepIUMPRFaultDetect.c');port_label('input',1,'RatioId');port_label('output',1,'ok');
  Terminator3 : Terminator
  wires:
  Dem_RepIUMPRFaultDetect/1 -> Terminator3/1
  Vc09/1 -> Dem_RepIUMPRFaultDetect/1
